simulink model "mcb_host_model_f28069m"  (R2021b)
settings: Solver=FixedStepDiscrete  StartTime=0.0  StopTime=inf  RelTol=1e-3  EnableMultiTasking=on
undefined symbols (not defined in the file or in its folder): PU_System, Ts
libraries: mcbhostblockslib x3
settings Model: Creator=The MathWorks, Inc.  LastModifiedBy=The MathWorks, Inc.
settings SolverCC: AlgebraicLoopSolver=TrustRegion
settings DataIOCC: LimitDataPoints=on  SaveFormat=Array  ReturnWorkspaceOutputs=off
settings OptimizationCC: LifeSpan=1  EfficientTunableParamExpr=on
settings DebuggingCC: UnderspecifiedInitializationDetection=Classic  MergeDetectMultiDrivingBlocksExec=none  SolverPrmCheckMsg=warning  ParameterPrecisionLossMsg=none  AllowSymbolicDim=off  PregeneratedLibrarySubsystemCodeDiagnostic=none  SFUnexpectedBacktrackingDiag=warning  SFNoUnconditionalDefaultTransitionDiag=warning  SFExecutionAtInitializationDiag=none  SFMachineParentedDataDiag=warning  ArithmeticOperatorsInVariantConditions=warning
settings HardwareCC: ProdBitPerPointer=32  ProdLargestAtomicFloat=None  ProdIntDivRoundTo=Undefined  ProdEndianess=Unspecified  ProdWordSize=32  ProdHWDeviceType=32-bit Generic
settings ModelReferenceCC: PropagateSignalLabelsOutOfModel=off
settings SFSimCC: SimUseLocalCustomCode=off  MATLABDynamicMemAlloc=off
settings RTWCC: Description=Real-Time Workshop Embedded Coder  SystemTargetFile=ert.tlc  TemplateMakefile=ert_default_tmf  GenerateReport=on  RTWUseLocalCustomCode=off  IncludeHyperlinkInReport=on  LaunchReport=on  GenerateTraceInfo=on  GenerateTraceReport=on  GenerateTraceReportSl=on  GenerateTraceReportSf=on  GenerateTraceReportEml=on
settings CodeAppCC: IgnoreCustomStorageClasses=off  StateflowObjectComments=on  InternalIdentifier=Classic
settings ERTTargetCC: MultiwordLength=2048  GenerateSampleERTMain=on  ERTCustomFileTemplate=example_file_process.tlc  ConvertIfToSwitch=off  SuppressUnreachableDefaultCases=off
settings ConfigComp: CovMetricSettings=dw  CovSaveCumulativeToWorkspaceVar=on  CovSaveSingleToWorkspaceVar=on  CovExternalEMLEnable=off  CovSFcnEnable=off

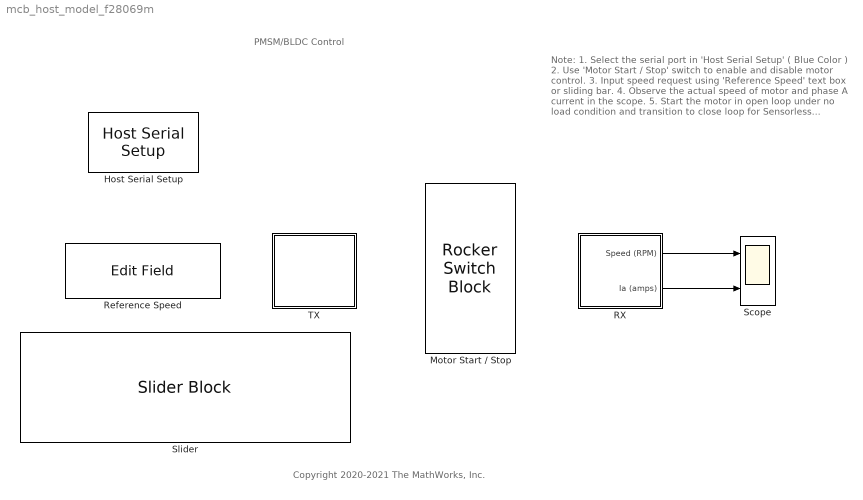
== system mcb_host_model_f28069m ==
  note: Copyright 2020-2021 The MathWorks, Inc.
  note: Note:
      | 1. Select the serial port in
      | 'Host Serial Setup' ( Blue Color )
      | 2. Use 'Motor Start / Stop' switch to enable and disable motor control.
      | 3. Input speed request using 'Reference Speed' text box or sliding bar.
      | 4. Observe the actual speed of motor and phase A current in the scope.
      | 5. Start the motor in open loop under no load condition and transition to close loop for Sensorless Example. The model works in open loop for speed ref below 0.1pu.
  note: PMSM/BLDC Control
  Host Serial Setup : mcbhostblockslib/Host Serial Setup  Priority=-99  comPortSer1='Please_select_a_port'  baudRateA=5.625e6  charLenA=8  stopBitA=1  parityA=none  timeoutA=2  ByteOrderA=LittleEndian  comPortSer2='Please_select_a_port'  baudRateB=115200  charLenB=8  stopBitB=1  parityB=none  timeoutB=1.0  ByteOrderB=LittleEndian  comPortSer3='Please_select_a_port'  baudRateC=115200  charLenC=8  stopBitC=1  parityC=none  timeoutC=1.0  ByteOrderC=LittleEndian  comPortSer4='Please_select_a_port'  baudRateD=115200  charLenD=8  stopBitD=1  parityD=none  timeoutD=1.0  ByteOrderD=LittleEndian
      settings: SourceProductBaseCode=MT
  Motor Start / Stop : RockerSwitchBlock  LabelPosition=Hide
      settings: Values={{'On', 'Off'}, [1 0]}
  RX : Subsystem
  Reference Speed : EditField  LabelPosition=Hide  ShowInitialText=on  Alignment=Center
  Scope : Scope  NumInputPorts=2
  Slider : SliderBlock  LabelPosition=Hide  ScaleMin=-6000  ScaleMax=6000
  TX : Subsystem
  wires:
  RX/1(Speed (RPM)) -> Scope/1
  RX/2(Ia (amps)) -> Scope/2

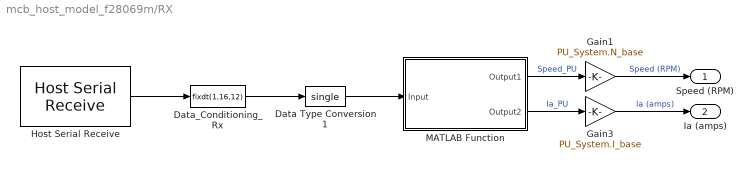
== system mcb_host_model_f28069m/RX ==
  Data Type Conversion1 : DataTypeConversion  OutDataTypeStr=single  RndMeth=Simplest
  Data_Conditioning_Rx : DataTypeConversion  OutDataTypeStr=fixdt(1,16,12)  ConvertRealWorld=Stored Integer (SI)  RndMeth=Simplest
  Gain1 : Gain  Gain=PU_System.N_base  OutDataTypeStr=single  RndMeth=Simplest
  Gain3 : Gain  Gain=PU_System.I_base  OutDataTypeStr=single  RndMeth=Simplest
  Host Serial Receive : mcbhostblockslib/Host Serial Receive  serialCon=Serial 1  dataHead='SS'  dataTail='EE'  dataType=uint16  dataDim=[600 2]  initValue=0  errOption=Output the last received value  errValue=0  sampleTime=600 * Ts  outputStatus=off  blockingMode=on
      settings: SourceProductBaseCode=MT
  MATLAB Function : MATLAB Function  TreatAsAtomicUnit=on
  Speed (RPM) : Outport
  Ia (amps) : Outport  Port=2
  wires:
  Data Type Conversion1/1 -> MATLAB Function/1(Input)
  Data_Conditioning_Rx/1 -> Data Type Conversion1/1
  Gain1/1 -> Speed (RPM)/1  "Speed (RPM)"
  MATLAB Function/1(Output1) -> Gain1/1  "Speed_PU"
  Host Serial Receive/1 -> Data_Conditioning_Rx/1
  Gain3/1 -> Ia (amps)/1  "Ia (amps)"
  MATLAB Function/2(Output2) -> Gain3/1  "Ia_PU"

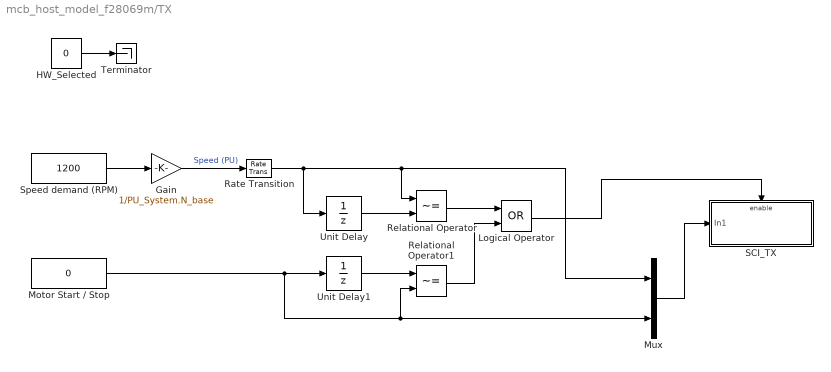
== system mcb_host_model_f28069m/TX ==
  Gain : Gain  Gain=1/PU_System.N_base  RndMeth=Simplest  OutDataTypeStr=Inherit: Same as input
  HW_Selected : Constant  Value=0  OutDataTypeStr=uint8
  Logical Operator : Logic  Operator=OR  AllPortsSameDT=off  OutDataTypeStr=boolean
  Motor Start / Stop : Constant  Value=0  VectorParams1D=off  OutDataTypeStr=single  SampleTime=0.03
  Mux : Mux  Inputs=2
  Rate Transition : RateTransition  OutPortSampleTime=0.03
  Relational Operator : RelationalOperator  Operator=~=  OutDataTypeStr=boolean  RndMeth=Nearest
  Relational Operator1 : RelationalOperator  Operator=~=  OutDataTypeStr=boolean  RndMeth=Nearest
  SCI_TX : Subsystem  TreatAsAtomicUnit=on
  Speed demand (RPM) : Constant  Value=1200  VectorParams1D=off  OutDataTypeStr=single  SampleTime=0.03
  Terminator : Terminator
  Unit Delay : UnitDelay  InitialCondition=0.5  SampleTime=-1  HasFrameUpgradeWarning=on
  Unit Delay1 : UnitDelay  SampleTime=-1  HasFrameUpgradeWarning=on
  wires:
  Motor Start / Stop/1 -> Relational Operator1/2, Mux/2, Unit Delay1/1
  Logical Operator/1 -> SCI_TX/Enable
  Rate Transition/1 -> Unit Delay/1, Mux/1, Relational Operator/1
  Mux/1 -> SCI_TX/1(In1)
  Speed demand (RPM)/1 -> Gain/1
  Gain/1 -> Rate Transition/1  "Speed (PU)"
  Relational Operator/1 -> Logical Operator/1
  Unit Delay/1 -> Relational Operator/2
  Relational Operator1/1 -> Logical Operator/2
  Unit Delay1/1 -> Relational Operator1/1
  HW_Selected/1 -> Terminator/1

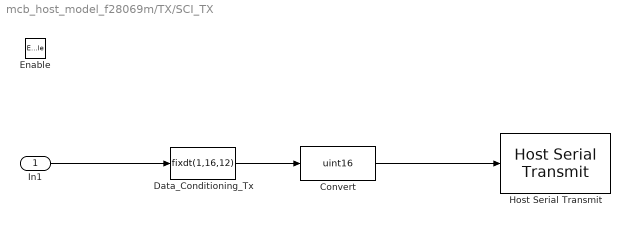
== system mcb_host_model_f28069m/TX/SCI_TX ==
  In1 : Inport
  Enable : EnablePort
  Convert : DataTypeConversion  OutDataTypeStr=uint16  ConvertRealWorld=Stored Integer (SI)  RndMeth=Simplest
  Data_Conditioning_Tx : DataTypeConversion  OutDataTypeStr=fixdt(1,16,12)  RndMeth=Simplest
  Host Serial Transmit : mcbhostblockslib/Host Serial Transmit  serialCon=Serial 1  header=''  tail=''  enableBlockingMode=off
      settings: SourceProductBaseCode=MT
  wires:
  Convert/1 -> Host Serial Transmit/1
  Data_Conditioning_Tx/1 -> Convert/1
  In1/1 -> Data_Conditioning_Tx/1

== matlab function mcb_host_model_f28069m/RX/MATLAB Function ==
  data: Output1 output; Output2 output; Input input
function [ Output1, Output2] = unBuf(Input)

Output1 = Input(:, 1);
Output2 = Input(:, 2);
end
